simulink library "hrc"  (Simulink 8.1)
settings: Solver=ode1  StartTime=0.0  StopTime=Inf  FixedStep=0.001  RelTol=1e-3
PostLoadFcn:
  | , if any(exist('dsrtsu_mdlpostloadfcn', 'file') == [2, 3, 6]), try dsrtsu_mdlpostloadfcn('Execute', bdroot); catch fprintf('Error in PostLoadFcn (dsrtsu_mdlpostloadfcn) for model "%s":\n %s\n', bdroot, lasterr); end, end,
undefined symbols (not defined in the file or in its folder): KACC_HoldModeLimitDecel_mps2, KACC_HoldModeLimitSpeed_kph
settings Model: DSRTSU_INTERNAL_RTI_VER=450  DSRTSU_INTERNAL_RTI_TYPE=rti1401  RTICANMMDATA=struct('GeneralSetupData',struct('modelroot','D:\ELN150201_TAIWAN\trunk\AdasDragon\software\sw_development\arch\app\acc','generalsettings',struct('filesettings',struct('destfolder',struct('Name','RTICANMM_FILES','Check',1),'buildfolder',struct('Name','.','Check',1),'AbsDestfolder',struct('Name','D:\ELN150201_TAIWAN\trunk\AdasDragon\software\sw_development\arch\app\acc\RTICANMM_FILES'),'AbsBuildfolder',struct('Name','D:\ELN150201_TAIWAN\trunk\AdasDragon\software\sw_development\arch\app\acc'))),'options',struct('addpaths',1,'rmpaths',1,'addtrcexclusion',logical(1),'cannavigator',struct('checkmonitoring',0),'show_usrtrc',0,'use_usrtrc',0),'advanced',struct('options',[1 1 1 1 1 1 1 1 1 1 1 1 1 1 1 1 1 1 1 1 1 1 1 1 1 1 1 1 1 1 1 1 1 1 1 1 1 1 1 1 1 1 1 1 1 1 1 1 1 1 1 1 1 1 1 1 1 1 1 1 1 1 1 1 1 1 1 1 1 1 1 1 1 1 1 1 1 1 1 1 1 1 1 1 1 1 1 1 1 1 1 1 1 1 1 1 1 1 1 1]),'MPSetup',{{}},'modelname','hrc','block','hrc'))  DSRTSU_INTERNAL_RTIFPGA=40  Creator=AT015411  LastModifiedBy=AT015555

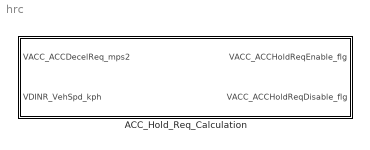
== system hrc ==
  ACC_Hold_Req_Calculation : Subsystem

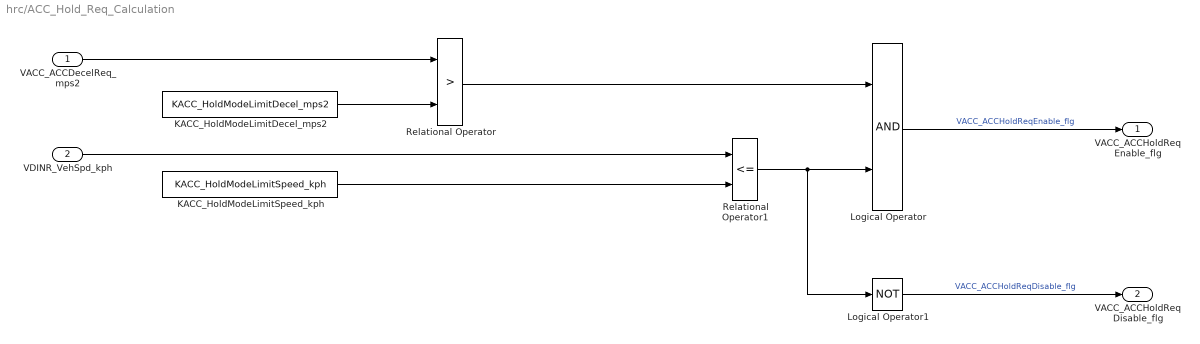
== system hrc/ACC_Hold_Req_Calculation ==
  VACC_ACCDecelReq_mps2 : Inport
  VDINR_VehSpd_kph : Inport  Port=2
  KACC_HoldModeLimitDecel_mps2 : Constant  Value=KACC_HoldModeLimitDecel_mps2
  KACC_HoldModeLimitSpeed_kph : Constant  Value=KACC_HoldModeLimitSpeed_kph
  Logical Operator : Logic  AllPortsSameDT=off  OutDataTypeStr=boolean
  Logical Operator1 : Logic  Operator=NOT  AllPortsSameDT=off  OutDataTypeStr=boolean
  Relational Operator : RelationalOperator  Operator=>  OutDataTypeStr=boolean
  Relational Operator1 : RelationalOperator  Operator=<=  OutDataTypeStr=boolean
  VACC_ACCHoldReqEnable_flg : Outport
  VACC_ACCHoldReqDisable_flg : Outport  Port=2
  wires:
  KACC_HoldModeLimitSpeed_kph/1 -> Relational Operator1/2
  Relational Operator1/1 -> Logical Operator1/1, Logical Operator/2
  VDINR_VehSpd_kph/1 -> Relational Operator1/1
  VACC_ACCDecelReq_mps2/1 -> Relational Operator/1
  Logical Operator/1 -> VACC_ACCHoldReqEnable_flg/1  "VACC_ACCHoldReqEnable_flg"
  KACC_HoldModeLimitDecel_mps2/1 -> Relational Operator/2
  Relational Operator/1 -> Logical Operator/1
  Logical Operator1/1 -> VACC_ACCHoldReqDisable_flg/1  "VACC_ACCHoldReqDisable_flg"
